simulink model "peacockElettricaSimulink"  (R2026a)
settings: Solver=FixedStepAuto  StopTime=40  FixedStep=0.001  EnableMultiTasking=on
InitFcn:
  | run('setupParams.m');
  | %run("tracks\track2.m");
StopFcn:
  | plot(out.X, out.Y);
  | axis equal;
  | grid on;
model workspace: external: MATLAB File (data not in the file)
values from neighbouring files (symbols this model uses):
  aero_bal_r = 0.5    [setupParams.m]    (also in setupParamsSingle.m)
  Af = 1.1    [setupParams.m]    (also in setupParamsSingle.m)
  auto_speed = 0    [setupParams.m]
  ay_limit = 15.0    (= 15)    [setupParams.m]    (also in setupParamsSingle.m)
  brake_bias_f = 0.40    (= 0.4)    [setupParams.m]    (also in setupParamsSingle.m = 0.6)
  brake_bias_r = 1 - brake_bias_f    (= 0.6)    [setupParams.m]    (also in setupParamsSingle.m = 0.4)
  camber_front = -1.5    [setupParams.m]    (also in setupParamsSingle.m)
  camber_rear = -1    [setupParams.m]    (also in setupParamsSingle.m)
  Cl = 1.0    (= 1)    [setupParams.m]    (also in setupParamsSingle.m)
  deathzone_APP = 5    [setupParams.m]    (also in setupParamsSingle.m)
  e_yaw_deadzone = 0.03    [setupParams.m]
  falling_slew_rate_torque = -500    [setupParams.m]    (also in setupParamsSingle.m)
  g = 9.81    [setupParams.m]    (also in setupParamsSingle.m)
  gnd_displ = 0.0    (= 0)    [setupParams.m]    (also in setupParamsSingle.m)
  h_o = 0.35    [setupParams.m]    (also in setupParamsSingle.m)
  I_charge_max = 21    [setupParams.m]
  I_discharge_max = 90    [setupParams.m]
  K_roll_rear = 0.6    [setupParams.m]    (also in setupParamsSingle.m = 0.5)
  Kus = 0.03    [setupParams.m]    (also in setupParamsSingle.m = 0)
  l_f = 0.775    [setupParams.m]    (also in setupParamsSingle.m)
  l_r = 0.775    [setupParams.m]    (also in setupParamsSingle.m)
  launch_ramp_rate = 1000.0    (= 1000)    [setupParams.m]    (also in setupParamsSingle.m)
  launch_V_thresh = 5.0    (= 5)    [setupParams.m]    (also in setupParamsSingle.m)
  mass = 320    [setupParams.m]    (also in setupParamsSingle.m = 300)
  mu = 1.5    [setupParams.m]    (also in setupParamsSingle.m)
  nominal_ramp_rate = 1000.0    (= 1000)    [setupParams.m]    (also in setupParamsSingle.m)
  overslip_factor = 1.01    [setupParams.m]    (also in setupParamsSingle.m = 1.13)
  pa_front_wheel = 82700    [setupParams.m]    (also in setupParamsSingle.m)
  pa_rear_wheel = 82700    [setupParams.m]    (also in setupParamsSingle.m)
  pedal_bp = (0:10:100)'    [setupParams.m]    (also in setupParamsSingle.m)
  pedal_map = (pedal_bp / 100) .^ pedal_alpha    [setupParams.m]    (also in setupParamsSingle.m = (pedal_bp / 100) .^ pedal_alpha.Value)
  R_wheel = 0.2032    [setupParams.m]    (also in setupParamsSingle.m)
  regen_I_cont_A = 14.0    (= 14)    [setupParams.m]    (also in setupParamsSingle.m)
  regen_I_peak_A = 21.0    (= 21)    [setupParams.m]    (also in setupParamsSingle.m)
  regen_I_peak_dur_s = 4.0    (= 4)    [setupParams.m]    (also in setupParamsSingle.m)
  regen_P_batt_max_W = 35000    [setupParams.m]    (also in setupParamsSingle.m)
  regen_pedal_thr = 5.0    (= 5)    [setupParams.m]    (also in setupParamsSingle.m = 10)
  regen_speed_crit_rpm = 1000    [setupParams.m]    (also in setupParamsSingle.m = 500)
  regen_speed_min_rpm = 4000    [setupParams.m]    (also in setupParamsSingle.m = 3000)
  regen_T_max = 9    [setupParams.m]    (also in setupParamsSingle.m = Simulink.Parameter(T_rated.Value/2))
  rho = 1.225    [setupParams.m]    (also in setupParamsSingle.m)
  rid_eff = 0.80    (= 0.8)    [setupParams.m]    (also in setupParamsSingle.m)
  rid_ratio = 15    [setupParams.m]    (also in setupParamsSingle.m)
  rising_slew_rate_torque = 100    [setupParams.m]    (also in setupParamsSingle.m)
  rpm_safe_threshold = 100    [setupParams.m]
  scale_factor_front = ones(27, 1)    [setupParams.m]    (also in setupParamsSingle.m)
  scale_factor_rear = ones(27, 1)    [setupParams.m]    (also in setupParamsSingle.m)
  slip_bc_coeff = 10    [setupParams.m]    (also in setupParamsSingle.m = Simulink.Parameter(1.5))
  slip_filt_N = 80    [setupParams.m]    (also in setupParamsSingle.m = 15)
  slip_Kd = 0.8    [setupParams.m]    (also in setupParamsSingle.m = Simulink.Parameter(5.0))
  slip_Ki = 13.0    (= 13)    [setupParams.m]    (also in setupParamsSingle.m = Simulink.Parameter(110.0))
  slip_Kp = 50.0    (= 50)    [setupParams.m]    (also in setupParamsSingle.m = Simulink.Parameter(180.0))
  slip_low_sat = 0.0    (= 0)    [setupParams.m]    (also in setupParamsSingle.m)
  slip_ref = 0.15    [setupParams.m]    (also in setupParamsSingle.m = Simulink.Parameter(0.15))
  slip_up_sat = 25    [setupParams.m]    (also in setupParamsSingle.m = 21)
  slip_V_min = 3    [setupParams.m]    (also in setupParamsSingle.m = 1)
  steer_ratio = 4.2    [pure_pursuit.m]    (also in setupParams.m; setupParamsSingle.m)
  steering_deadband = 1    [setupParams.m]
  T_headroom_k = 13.0    (= 13)    [setupParams.m]    (also in setupParamsSingle.m = Simulink.Parameter(5.0))
  T_headroom_max = 9    [setupParams.m]    (also in setupParamsSingle.m = Simulink.Parameter(5.0))
  T_peak = 20    [setupParams.m]    (also in setupParamsSingle.m = 21)
  T_rated = 9.8    [setupParams.m]    (also in setupParamsSingle.m = Simulink.Parameter(9.8))
  track_width = (track_width_r + track_width_f)/2    (= 1.2)    [setupParams.m]    (also in setupParamsSingle.m = sqrt(track_width_r^2 + track_width_f^2))
  track_width_f = 1.2    [setupParams.m]    (also in setupParamsSingle.m)
  track_width_r = 1.2    [setupParams.m]    (also in setupParamsSingle.m)
  Ts = 0.01    [setupParams.m]    (also in setupParamsSingle.m)
  tvc_bc = 17    [setupParams.m]
  tvc_D_thresh = 0.060    (= 0.06)    [setupParams.m]    (also in setupParamsSingle.m)
  tvc_D_thresh_off = 0.03    [setupParams.m]    (also in setupParamsSingle.m)
  tvc_Kd = 100    [setupParams.m]    (also in setupParamsSingle.m = Simulink.Parameter(5))
  tvc_Ki = 150    [setupParams.m]    (also in setupParamsSingle.m = Simulink.Parameter(10))
  tvc_Kp = 650    [setupParams.m]    (also in setupParamsSingle.m = Simulink.Parameter(70))
  tvc_N_filter = 25    [setupParams.m]    (also in setupParamsSingle.m = Simulink.Parameter(20))
  tvc_sat_dMz = 700    [setupParams.m]    (also in setupParamsSingle.m = Simulink.Parameter(10.0))
  tvc_throttle_on = 3.0    (= 3)    [setupParams.m]    (also in setupParamsSingle.m = Simulink.Parameter(3.0))
  tvc_tr = 5    [setupParams.m]    (also in setupParamsSingle.m = Simulink.Parameter(1.0))
  tvc_V_off = 2.0    (= 2)    [setupParams.m]    (also in setupParamsSingle.m = Simulink.Parameter(2.0))
  tvc_V_on = 4.0    (= 4)    [setupParams.m]    (also in setupParamsSingle.m = Simulink.Parameter(4.0))
  tvc_yaw_thresh = 0.08    [setupParams.m]    (also in setupParamsSingle.m)
  tvc_yaw_thresh_off = 0.04    [setupParams.m]    (also in setupParamsSingle.m)
  V_dc = 540    [setupParams.m]    (also in setupParamsSingle.m)
  w_engine = 0.005    [setupParams.m]    (also in setupParamsSingle.m)
  wheelbase = l_f + l_r    (= 1.55)    [setupParams.m]    (also in setupParamsSingle.m)
undefined symbols (not defined in the file or in its folder): V_ref, X_ref, Y_ref
libraries: simulink x74, slpidlib x8, vehdynlibtire x8, dspsigops x4, vehdynlibsteering x2, autolibshared x2, sim3dautolib x2, sim3dlib x1, robotalgslib x1
(part 1 of 6)
settings Model: SimulationMode=accelerator  SILPILModeSetting=veronly  ExtModeTrigDuration=10  Creator=Utente  LastModifiedBy=Utente
settings SolverCC: ZeroCrossControl=DisableAll  PositivePriorityOrder=on  EnableFixedStepZeroCrossing=on
settings DataIOCC: SaveFormat=StructureWithTime
settings OptimizationCC: BufferReuse=off
settings DebuggingCC: AlgebraicLoopMsg=error  MultiTaskRateTransMsg=warning
settings HardwareCC: ProdLargestAtomicInteger=Long  ProdLargestAtomicFloat=Double  ProdHWDeviceType=ARM Compatible->ARM Cortex-M  TargetLargestAtomicInteger=Long  TargetLargestAtomicFloat=Float  TargetIntDivRoundTo=Zero  TargetEndianess=LittleEndian  TargetHWDeviceType=ARM Compatible->ARM 10
settings ModelReferenceCC: ModelReferenceNumInstancesAllowed=Single
settings RTWCC: SystemTargetFile=ert.tlc  HardwareBoard=STM32G4xx Based  TLCOptions=-aInlineSetEventsForThisBaseRateFcn=TLC_FALSE -aSuppressMultiTaskScheduler=TLC_FALSE -aRateBasedStepFcn=1  GenCodeOnly=on  Toolchain=GNU Tools for STM32  BuildConfiguration=Faster Runs  Description=Embedded Coder
settings ERTTargetCC: ExtModeTransport=3.0  ExtModeStaticAllocSize=2048.0  CodeReplacementLibrary=ARM Cortex-M  SubcomponentCodeInterfacePackaging=Nonreusable function

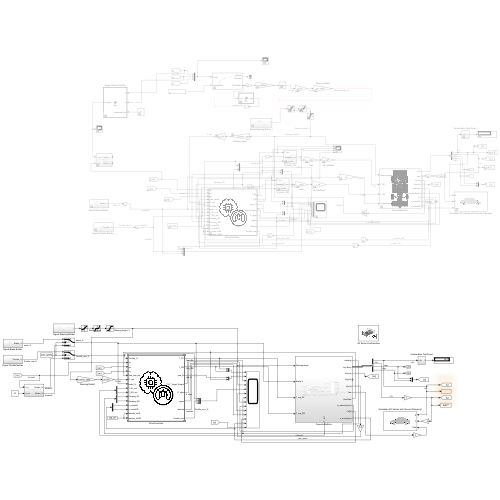
[thumbnail: Simulink's stored preview of the top-level diagram]
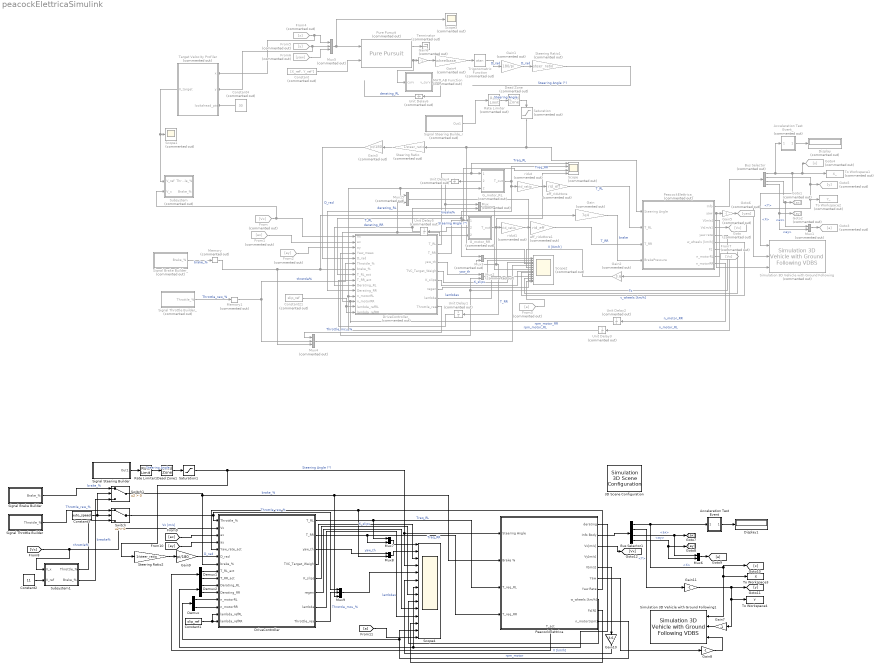
== system peacockElettricaSimulink ==
  " 3D Scene Configuration" : sim3dlib/Simulation 3D Scene Configuration  Priority=0  ProjectFormat=Default Scenes  SceneDesc=Open surface  ProjectName=Z:\.Programmi\MATLAB26a\toolbox\shared\sim3d_projects\automotive_project_windows\UE\WindowsNoEditor\VehicleSimulation.exe  ScenePath=/Game/Maps/HwStrght  EnableOpenDRIVE=off  vehTagList={'Custom';'Scene Origin';'SimulinkVehicle1';'SimulinkVehicle2'}  vehTag=SimulinkVehicle2  AttachedCameraRelativeTranslation=[0 0 0]  FreeCameraDefaultInitialTranslation=[-6, 0, 2]  AttachedCameraRelativeRotation=[0 0 0]  FreeCameraDefaultInitialRotation=[0, -15, 0]  ViewpointName=Custom  FreeCameraInitialTranslation=[0 0 0]  FreeCameraInitialRotation=[0 0 0]  OpVisEn=off  Ts=.03  EnableWindow=off  EnableRemoteAccess=off  SimulationMode=CoSimulation  SimulateUsing=Interpreted execution  EnableAnimationRecording=off  OverrideDefaultRecording=off  AnimationRecordingFileName=sim3dAnimation.mat  AnimationRecordingInterval=[0 inf]  EnableWeather=off  SunAzimuth=90  SunAltitude=40.0  EnableGeospatialSun=off  Latitude=0  Longitude=0  Date=2023-01-01  Time=10:30:00  GeoTimeZone=-5.0  SunDaylightSaving=off  wind=1  clouds=10  EnableVolumetricClouds=off  CloudCoverage=0  CloudAltitude=6  fog=0  rain=0  RaindropsEffect=off  SnowDensity=0  EnableGeospatial=off  TilesetSource=Earth terrain  UseTrueOrigin=off  OriginHeight=200  OriginLatitude=40.744652  OriginLongitude=-73.988864  MapStyle=Aerial  AdditionalAssetIDs=[]  UseAdvancedSunSky=off  SolarTime=11  TimeZone=-5  Day=21  Month=9  Year=2022  UseDaylightSavingTime=on  DSTStartDay=10  DSTStartMonth=3  DSTEndDay=3  DSTEndMonth=11  DSTSwitchHour=2  sensorTag=MainCamera1  sensorId=1  sensorName=MainCamera1  mountLoc=Origin  offsetFlag=off  tmountOffset=[0, 0, 0]  rmountOffset=[0, 0, 0]  HorizontalResolution=1280  VerticalResolution=720  HorizontalFOV=60  mountPoint=[0 0 0]  mountOrientation=[0 0 0]  aMode=2  ID=1  GeoTrigger=Inactive  ViewNameList={'Custom'}  ViewTranslationList={'[0 0 0]'}  ViewRotationList={'[0 0 0]'}
      settings: LibrarySourceBlock=vehdynlibsim3dcore/Simulation 3D Scene Configuration
  Acceleration Test Event : Subsystem
  Acceleration Test Event_ : Subsystem  Commented=on
  Bus Selector : BusSelector  Commented=on  OutputSignals=InertFrm.Geom.Disp.X,InertFrm.Geom.Disp.Y,BdyFrm.Cg.Acc.ax,BdyFrm.Cg.Acc.ay
  Bus Selector1 : BusSelector  OutputSignals=InertFrm.Geom.Disp.X,InertFrm.Geom.Disp.Y,BdyFrm.Cg.Acc.ax,BdyFrm.Cg.Acc.ay
  Constant : Constant  Commented=on  Value=[X_ref', Y_ref']
  Constant1 : Constant  Value=slip_ref
  Constant2 : Constant  Value=11
  Constant21 : Constant  Commented=on  Value=slip_ref
  Constant3 : Constant  Value=auto_speed
  Constant4 : Constant  Commented=on  Value=30
  Dead Zone : DeadZone  Commented=on  LowerValue=-2  UpperValue=2
  Dead Zone1 : DeadZone  LowerValue=-2  UpperValue=2
  Demux : Demux  Outputs=2
  Demux1 : Demux  Outputs=2
  Demux2 : Demux  Outputs=2
  Display : Display  Commented=on
  Display1 : Display
  DriveController : Subsystem  TreatAsAtomicUnit=on
      mask Display: image('smart_14958016.png', [0,0,0,0,60,60]);
  DriveController_ : Subsystem  Commented=on  TreatAsAtomicUnit=on
      mask Display: image('smart_14958016.png', [0,0,0,0,60,60]);
  From : From  Commented=on  GotoTag=Vx
  From1 : From  Commented=on  GotoTag=ax
  From2 : From  Commented=on  GotoTag=ay
  From3 : From  Commented=on  GotoTag=a
  From4 : From  Commented=on  GotoTag=x
  From5 : From  Commented=on  GotoTag=y
  From6 : From  Commented=on  GotoTag=yaw
  From7 : From  Commented=on  GotoTag=Vx
  G_motor_RL : Subsystem  Commented=on
      settings: PortSchema="{\"entries\":[{\"content\":{\"sides\":[{\"content\":{\"connectorIds\":[\"In1\",\"Out2\",\"In2\"]},\"type\":\"ConnectorPlacement.EquallySpacedRectSide\",\"uuid\":\"2f848e13-22e7-46a8-96e7-944fd1b36019\"},{\"content\":{\"connectorIds\":[\"Out1\"],\"side\":\"RIGHT\"},\"type\":\"ConnectorPlacement.EquallySpacedRectSide\",\"uuid\":\"64718f6e-925f-4c2e-9ed1-674a318236f8\"},{\"content\":{\"side\":\"TOP\"},\"type\":\"ConnectorPlacement.EquallySpacedRectSide\",\"uuid\":\"f53d168c-fae3-4286-a18b-c9c25d6ee575\"}]},\"type\":\"ConnectorPlacement.EquallySpacedConnector\",\"uuid\":\"bc8637a2-640e-4920-833f-efe601435780\"}],\"packageUris\":[\"http://schema.mathworks.com/mf0/Connector/R2020b\"],\"version\":\"1.0\"}"
  G_motor_RR : Subsystem  Commented=on
      settings: PortSchema="{\"entries\":[{\"content\":{\"sides\":[{\"content\":{\"connectorIds\":[\"In1\",\"Out2\",\"In2\"]},\"type\":\"ConnectorPlacement.EquallySpacedRectSide\",\"uuid\":\"b35581c9-4812-43f6-acf6-85982729658e\"},{\"content\":{\"connectorIds\":[\"Out1\"],\"side\":\"RIGHT\"},\"type\":\"ConnectorPlacement.EquallySpacedRectSide\",\"uuid\":\"46b9f9af-9e32-4108-a19f-3f2988ef12f0\"},{\"content\":{\"side\":\"TOP\"},\"type\":\"ConnectorPlacement.EquallySpacedRectSide\",\"uuid\":\"065300c1-2443-4807-8b2c-2500fecbac33\"}]},\"type\":\"ConnectorPlacement.EquallySpacedConnector\",\"uuid\":\"282786dd-8e40-401f-94f1-60a6482c0151\"}],\"packageUris\":[\"http://schema.mathworks.com/mf0/Connector/R2020b\"],\"version\":\"1.0\"}"
  Gain : Gain  Commented=on  Gain=7e4
  Gain1 : Gain  Commented=on  Gain=180/pi
  Gain10 : Gain  Gain=3.6
  Gain11 : Gain  Gain=-1
  Gain2 : Gain  Commented=on  Gain=3.6
  Gain3 : Gain  Commented=on  Gain=pi/180
  Gain4 : Gain  Commented=on  Gain=wheelbase
  Gain5 : Gain  Commented=on  Gain=-1
  Gain6 : Gain  Commented=on  Gain=-1
  Gain7 : Gain  Gain=-1
  Gain8 : Gain  Gain=-1
  Gain9 : Gain  Gain=pi/180
  Goto : Goto  Commented=on  GotoTag=Vx
  Goto1 : Goto  Commented=on  GotoTag=ax
  Goto2 : Goto  Commented=on  GotoTag=ay
  Goto3 : Goto  Commented=on  GotoTag=a
  Goto4 : Goto  Commented=on  GotoTag=x
  Goto5 : Goto  Commented=on  GotoTag=y
  Goto6 : Goto  Commented=on  GotoTag=yaw
  MATLAB Function : MATLAB Function  Commented=on  TreatAsAtomicUnit=on
  Memory : Memory  Commented=on
  Memory1 : Memory  Commented=on
  Mux{,1..3,15} (5 alike) : Mux  Commented=on  Inputs=2
  Mux4 : Mux  Commented=on  Inputs=3
  Mux5 : Mux  Commented=on  Inputs=3
  Mux6 : Mux  Inputs=2
  Mux7 : Mux  Inputs=2
  Mux8 : Mux  Inputs=2
  Mux9 : Mux  Inputs=3
  PeacockElettrica : Subsystem
      settings: PortSchema="{\"entries\":[{\"content\":{\"sides\":[{\"content\":{\"connectorIds\":[\"In1\",\"In2\",\"In3\",\"In4\"]},\"type\":\"ConnectorPlacement.EquallySpacedRectSide\",\"uuid\":\"9482d8e6-6871-478e-8a9d-73044ed7ab0e\"},{\"content\":{\"connectorIds\":[\"Out1\",\"Out2\",\"Out3\",\"Out4\",\"Out5\",\"Out6\",\"Out7\",\"Out8\",\"Out9\",\"Out10\"],\"side\":\"RIGHT\"},\"type\":\"ConnectorPlacement.EquallySpacedRectSide\",\"uuid\":\"cce15458-935a-453b-a26c-3a0c8875c305\"},{\"content\":{\"side\":\"TOP\"},\"type\":\"ConnectorPlacement.EquallySpacedRectSide\",\"uuid\":\"47cf2278-8524-4513-ad68-abd8f65e3014\"},{\"content\":{\"connectorIds\":[\"Out11\"],\"side\":\"BOTTOM\"},\"type\":\"ConnectorPlacement.EquallySpacedRectSide\",\"uuid\":\"d42c0be2-8d27-4d2e-97e3-233d61a32782\"}]},\"type\":\"ConnectorPlacement.EquallySpacedConnector\",\"uuid\":\"48bc61f2-5937-4956-9c2e-81c9fcf139cd\"}],\"packageUris\":[\"http://schema.mathworks.com/mf0/Connector/R2020b\"],\"version\":\"1.0\"}"
  PeacockElettrica_ : Subsystem  Commented=on
      mask Display: image('car.png', [0,0,0,0,60,100]);
  Pure Pursuit : robotalgslib/Pure Pursuit  Commented=on  DesiredLinearVelocityPort=off  DesiredLinearVelocity=0.1  MaxCurvature=1.0  LookaheadDistancePort=off  LookaheadDistance=1.5  TargetDirPort=off  SimulateUsing=Code generation
      settings: LibrarySourceBlock=navlib/Control Algorithms/Pure Pursuit
  Rate Limiter : RateLimiter  Commented=on  RisingSlewLimit=150  FallingSlewLimit=-150  SampleTimeMode=inherited
  Rate Limiter1 : RateLimiter  RisingSlewLimit=150  FallingSlewLimit=-150  SampleTimeMode=inherited
  Saturation : Saturate  Commented=on  UpperLimit=130  LowerLimit=-130
  Saturation1 : Saturate  UpperLimit=130  LowerLimit=-130
  Scope : Scope  Commented=on  NumInputPorts=4
      settings: ActiveDisplayYMinimum=-1.6967488885152928  ActiveDisplayYMaximum=15.270739996637639  DataLoggingVariableName=ScopeData5
  Scope1 : Scope  Commented=on
      settings: ActiveDisplayYMinimum=14.39563708692528  ActiveDisplayYMaximum=39.921268336925294  DataLoggingVariableName=ScopeData3
  Scope2 : Scope  Commented=on  NumInputPorts=14
      settings: AxesScalingNumUpdates=20  ActiveDisplayYMinimum=-11.688915556246606  ActiveDisplayYMaximum=16.101237530940978  DataLoggingVariableName=ScopeData2
  Scope3 : Scope  Commented=on
      settings: DataLoggingVariableName=ScopeData6
  Scope4 : Scope  NumInputPorts=14
      settings: ActiveDisplayYMinimum=-2.909562920832391  ActiveDisplayYMaximum=18.107750958840505  DataLoggingVariableName=ScopeData7
  Signal Brake Builder : Subsystem
  Signal Brake Builder_ : Subsystem  Commented=on
  Signal Steering Builde_r : Subsystem  Commented=on
  Signal Steering Builder : Subsystem
  Signal Throttle Builder : Subsystem
  Signal Throttle Builder_ : Subsystem  Commented=on
  Simulation 3D Vehicle with Ground Following : sim3dautolib/Simulation 3D Vehicle with Ground Following VDBS  Priority=-1  Commented=on  PassVehMesh=Formula student vehicle  MeshPath=/MathWorksAutomotiveContent/Vehicles/Muscle/Meshes/SK_MuscleCar.SK_MuscleCar  TrackWidth=1.9  WheelBase=3  WheelRadius=0.35  VehColor=Red  CoordinateSystem=SAE  InitialPos=[0, 0, 0]  InitialRot=[0,0,0]  ActorName=SimulinkVehicle1  VehLightsControl=off  HeadlightColor=[ 1, 1, 1 ]  HighBeamIntensity=100000  LowBeamIntensity=60000  HighBeamConeAngle=1.22  LowBeamConeAngle=1.22  LeftHeadlightOrientation=[ 0, 0 ]  RightHeadlightOrientation=[ 0, 0 ]  BrakelightIntensity=200  ReverselightIntensity=500  SignallightIntensity=500  SignallightPeriod=1  SignalPulseWidth=50  SampleTime=-1  ActorType=SimulinkVehicle  ID=1  aMode=2  ActorTag=SimulinkVehicle1  CoordinateScheme=0
      settings: LibrarySourceBlock=vehdynlibsim3d/Simulation 3D Vehicle with Ground Following
  Simulation 3D Vehicle with Ground Following1 : sim3dautolib/Simulation 3D Vehicle with Ground Following VDBS  Priority=-1  PassVehMesh=Formula student vehicle  MeshPath=/MathWorksAutomotiveContent/Vehicles/Muscle/Meshes/SK_MuscleCar.SK_MuscleCar  TrackWidth=1.9  WheelBase=3  WheelRadius=0.35  VehColor=Red  CoordinateSystem=SAE  InitialPos=[0, 0, 0]  InitialRot=[0,0,0]  ActorName=SimulinkVehicle2  VehLightsControl=off  HeadlightColor=[ 1, 1, 1 ]  HighBeamIntensity=100000  LowBeamIntensity=60000  HighBeamConeAngle=1.22  LowBeamConeAngle=1.22  LeftHeadlightOrientation=[ 0, 0 ]  RightHeadlightOrientation=[ 0, 0 ]  BrakelightIntensity=200  ReverselightIntensity=500  SignallightIntensity=500  SignallightPeriod=1  SignalPulseWidth=50  SampleTime=-1  ActorType=SimulinkVehicle  ID=2  aMode=2  ActorTag=SimulinkVehicle2  CoordinateScheme=0
      settings: LibrarySourceBlock=vehdynlibsim3d/Simulation 3D Vehicle with Ground Following
  Steering Ratio : Gain  Commented=on  Gain=1/steer_ratio
  Steering Ratio1 : Gain  Commented=on  Gain=steer_ratio
  Steering Ratio2 : Gain  Gain=1/steer_ratio
  Subsystem : Subsystem  Commented=on
  Subsystem1 : Subsystem
  Switch : Switch  Criteria=u2 > Threshold  SaturateOnIntegerOverflow=off  InputSameDT=off
  Switch1 : Switch  Criteria=u2 > Threshold  SaturateOnIntegerOverflow=off  InputSameDT=off
  Target Velocity Profiler : MATLAB Function  Commented=on  TreatAsAtomicUnit=on
  Terminator : Terminator  Commented=on
  To Workspace1 : ToWorkspace  Commented=on  VariableName=X_  SampleTime=0.05
  To Workspace2 : ToWorkspace  Commented=on  VariableName=Y_  SampleTime=0.05
  To Workspace3 : ToWorkspace  VariableName=X  SampleTime=0.05
  To Workspace4 : ToWorkspace  VariableName=Y  SampleTime=0.05
  Trigonometric Function : Trigonometry  Commented=on  Operator=atan
  Unit Delay{1..6} (6 alike) : UnitDelay  Commented=on  SampleTime=-1
  eff_riduttore : Gain  Commented=on  Gain=rid_eff
  eff_riduttore1 : Gain  Commented=on  Gain=rid_eff
  ridut : Gain  Commented=on  Gain=rid_ratio
  ridut1 : Gain  Commented=on  Gain=rid_ratio
  wires:
  G_motor_RL/1(T_out) -> Scope/2, DriveController_/8(T_RL_act), Mux3/1, ridut/1  "T_RL"
  Rate Limiter/1 -> Dead Zone/1  "Steering Angle"
  Saturation/1 -> PeacockElettrica_/1(Steering Angle), Scope2/4, Steering Ratio/1  "Steering Angle (°)"
  DriveController_/2(T_RR) -> Scope/3, G_motor_RR/1(T_req)  "Treq_RR"
  Bus Selector/1 -> Simulation 3D Vehicle with Ground Following/1, Goto4/1, To Workspace1/1, Acceleration Test Event_/1(<X>)  "<X>"
  eff_riduttore/1 -> PeacockElettrica_/2(T_RL)  "T_RL"
  Mux3/1 -> Scope2/1
  ridut1/1 -> eff_riduttore1/1
  ridut/1 -> eff_riduttore/1
  Steering Ratio/1 -> Gain3/1
  Bus Selector/2 -> Goto5/1, Simulation 3D Vehicle with Ground Following/2, To Workspace2/1  "<Y>"
  Dead Zone/1 -> Saturation/1
  G_motor_RR/1(T_out) -> Scope/4, Unit Delay1/1, Mux3/2, ridut1/1  "T_RR"
  Mux2/1 -> Scope2/2
  eff_riduttore1/1 -> PeacockElettrica_/3(T_RR)  "T_RR"
  DriveController_/1(T_RL) -> Scope/1, G_motor_RL/1(T_req)  "Treq_RL"
  PeacockElettrica_/5(yaw rate) -> DriveController_/4(Yaw_meas), Mux2/2
  Trigonometric Function/1 -> Gain1/1  "D_rad"
  Unit Delay1/1 -> DriveController_/9(T_RR_act)
  Unit Delay5/1 -> Mux/2, DriveController_/10(Derating_RL)  "derating_RR"
  G_motor_RL/2(derating) -> Unit Delay4/1
  DriveController_/3(yaw_th) -> Mux2/1  "yaw_th"
  DriveController_/4(TVC_Target_Weight) -> Scope2/3
  Mux/1 -> Scope2/7
  Signal Throttle Builder_/1(Throttle_%) -> Memory1/1  "Throttle_raw_%"
  Mux4/1 -> Scope2/5
  Constant21/1 -> DriveController_/14(lambda_refRL), DriveController_/15(lambda_refRR)
  DriveController_/5(K_slips) -> Scope2/8  "K_slips"
  DriveController_/6(regen) -> Scope2/10
  DriveController_/8(Throttle_real) -> Mux4/1  "Throttle_mcu_%"
  DriveController_/7(lambda) -> Scope2/11  "lambdas"
  Unit Delay4/1 -> Mux/1, DriveController_/11(Derating_RR)  "derating_RL"
  G_motor_RR/2(derating) -> Unit Delay5/1
  Mux15/1 -> Scope2/13
  PeacockElettrica_/8(n_motorRL) -> Unit Delay3/1  "n_motor_RL"
  PeacockElettrica_/9(n_motorRR) -> Unit Delay2/1  "n_motor_RR"
  PeacockElettrica_/1(Info) -> Bus Selector/1
  PeacockElettrica_/2(yaw) -> Gain5/1, Simulation 3D Vehicle with Ground Following/3
  PeacockElettrica_/3(V[m/s]) -> Gain2/1
  PeacockElettrica_/6(w_wheels [km/h]) -> Scope2/9  "v_wheels [km/h]"
  PeacockElettrica_/7(Fz) -> Scope2/12  "Fz"
  Gain2/1 -> Scope2/6  "V [Km/h]"
  PeacockElettrica_/4(Vx[m/s]) -> Goto/1
  From/1 -> Subsystem/2(V_x), DriveController_/1(Vx)
  From1/1 -> DriveController_/2(ax)
  Bus Selector/4 -> Goto2/1, Mux1/2  "<ay>"
  Bus Selector/3 -> Mux1/1, Goto1/1  "<ax>"
  From2/1 -> DriveController_/3(ay)
  Signal Brake Builder_/1(Brake_%) -> Memory/1  "brake_%"
  Acceleration Test Event_/1(Out1) -> Display/1
  Mux1/1 -> Goto3/1
  From3/1 -> Scope2/14
  Unit Delay2/1 -> G_motor_RR/2(rpm_motor), Mux15/2, DriveController_/13(n_motorRR)  "rpm_motor_RR"
  Unit Delay3/1 -> Mux15/1, G_motor_RL/2(rpm_motor), DriveController_/12(n_motorRL)  "rpm_motor_RL"
  Signal Steering Builde_r/1(Out1) -> Rate Limiter/1
  Gain/1 -> PeacockElettrica_/4(BrakePressure)  "brake"
  Mux5/1 -> Scope3/1, Pure Pursuit/1
  From4/1 -> Target Velocity Profiler/1(x), Mux5/1
  From5/1 -> Target Velocity Profiler/2(y), Mux5/2
  From6/1 -> Mux5/3
  Gain4/1 -> Trigonometric Function/1
  Constant/1 -> Pure Pursuit/2
  Gain1/1 -> Steering Ratio1/1  "D_rad"
  Gain3/1 -> DriveController_/5(D_rad)  "D_rad"
  Memory/1 -> Gain/1, DriveController_/7(brake_%), Mux4/3  "breake%"
  Memory1/1 -> DriveController_/6(Throttle_%), Mux4/2  "throttle%"
  Steering Ratio1/1 -> ?  "Steering Angle (°)"
  MATLAB Function/1(v_curv) -> Unit Delay6/1
  Unit Delay6/1 -> ?  "derating_RL"
  Gain5/1 -> Goto6/1
  Constant4/1 -> Target Velocity Profiler/3(lookahead_pts)
  Target Velocity Profiler/1(V_target) -> Scope1/1, Subsystem/1(V_ref)
  Pure Pursuit/1 -> Terminator/1
  Pure Pursuit/2 -> Gain6/1, MATLAB Function/1(curv)
  Gain6/1 -> Gain4/1
  DriveController/1(T_RL) -> Mux7/1, PeacockElettrica/3(T_req_RL)  "Treq_RL"
  DriveController/2(T_RR) -> Mux7/2, PeacockElettrica/4(T_req_RR)  "Treq_RR"
  Switch1/1 -> DriveController/7(brake_%), PeacockElettrica/2(Brake %), Mux9/3  "brake_%"
  Signal Steering Builder/1(Out1) -> Rate Limiter1/1
  Rate Limiter1/1 -> Dead Zone1/1  "Steering Angle"
  Dead Zone1/1 -> Saturation1/1
  Switch/1 -> Mux9/1, DriveController/1(Throttle_%)  "Throttle_raw_%"
  PeacockElettrica/10(n_motor[rpm]) -> Scope4/13, Demux/1  "rpm_motor"
  Demux/1 -> DriveController/12(n_motorRL)
  Demux/2 -> DriveController/13(n_motorRR)
  Constant1/1 -> DriveController/14(lambda_refRL), DriveController/15(lambda_refRR)
  PeacockElettrica/2(Info Body) -> Bus Selector1/1
  Bus Selector1/3 -> Mux6/1, [ax]  "<ax>"
  Bus Selector1/4 -> Mux6/2, [ay]  "<ay>"
  Mux6/1 -> [a]
  Bus Selector1/2 -> Gain11/1  "<Y>"
  PeacockElettrica/6(Yaw) -> Gain8/1
  Gain7/1 -> Simulation 3D Vehicle with Ground Following1/2
  Gain8/1 -> Simulation 3D Vehicle with Ground Following1/3
  Acceleration Test Event/1(Out1) -> Display1/1
  Bus Selector1/1 -> Acceleration Test Event/1(<X>), Simulation 3D Vehicle with Ground Following1/1, To Workspace3/1, [x]  "<X>"
  PeacockElettrica/3(Vx[m/s]) -> [Vx]
  [Vx] -> Subsystem1/1(V_x), DriveController/2(Vx)  "Vx [m/s]"
  PeacockElettrica/11(T_act) -> Demux1/1
  Demux1/1 -> DriveController/8(T_RL_act)
  Demux1/2 -> DriveController/9(T_RR_act)
  PeacockElettrica/1(derating) -> Scope4/7, Demux2/1
  Demux2/1 -> DriveController/10(Derating_RL)
  Demux2/2 -> DriveController/11(Derating_RR)
  PeacockElettrica/7(Yaw Rate) -> Mux8/2, DriveController/5(Yaw_rate_act)
  Saturation1/1 -> Steering Ratio2/1, PeacockElettrica/1(Steering Angle), Scope4/4  "Steering Angle (°)"
  Steering Ratio2/1 -> Gain9/1
  Gain9/1 -> DriveController/6(D_rad)  "D_rad"
  [ax] -> DriveController/3(ax)
  [ay] -> DriveController/4(ay)
  Mux7/1 -> Scope4/1
  DriveController/3(yaw_th) -> Mux8/1  "yaw_th"
  Mux8/1 -> Scope4/2
  DriveController/4(TVC_Target_Weight) -> Scope4/3
  DriveController/8(Throttle_real) -> Mux9/2  "Throttle_mcu_%"
  Mux9/1 -> Scope4/5
  PeacockElettrica/5(V[m/s]) -> Gain10/1
  Gain10/1 -> Scope4/6  "V [km/h]"
  DriveController/5(K_slips) -> Scope4/8  "K_slips"
  PeacockElettrica/8(w_wheels [km/h]) -> Scope4/9
  DriveController/6(regen) -> Scope4/10
  DriveController/7(lambda) -> Scope4/11  "lambdas"
  PeacockElettrica/9(Fz[N]) -> Scope4/12
  [a] -> Scope4/14
  Gain11/1 -> Gain7/1, To Workspace4/1, [y]
  Constant2/1 -> Subsystem1/2(V_ref)
  Signal Throttle Builder/1(Throttle_%) -> Switch/1  "Throttle_raw_%"
  Signal Brake Builder/1(Brake_%) -> Switch1/1  "brake_%"
  Subsystem1/1(Throttle_%) -> Switch/3  "throttle%"
  Subsystem1/2(Brake_%) -> Switch1/3  "breake%"
  Constant3/1 -> Switch1/2, Switch/2

== system peacockElettricaSimulink/Acceleration Test Event ==
  <X> : Inport
  Clock : Clock
  Clock1 : Clock
  Finish : HitCross  HitCrossingOffset=75.3  HitCrossingDirection=rising
  Sample and Hold : dspsigops/Sample and Hold  trig=Rising edge  initCond=0  latchinput=off
  Sample and Hold1 : dspsigops/Sample and Hold  trig=Rising edge  initCond=0  latchinput=off
  Start : HitCross  HitCrossingOffset=0.3  HitCrossingDirection=rising
  Sum : Sum  Inputs=|-+
  Out1 : Outport
  wires:
  Sample and Hold/1 -> Sum/2
  Sample and Hold1/1 -> Sum/1
  Finish/1 -> Sample and Hold/Trigger
  <X>/1 -> Finish/1, Start/1
  Clock1/1 -> Sample and Hold1/1
  Start/1 -> Sample and Hold1/Trigger
  Sum/1 -> Out1/1
  Clock/1 -> Sample and Hold/1

== system peacockElettricaSimulink/Acceleration Test Event_ ==
  <X> : Inport
  Clock : Clock
  Clock1 : Clock
  Finish : HitCross  HitCrossingOffset=75.3  HitCrossingDirection=rising
  Sample and Hold : dspsigops/Sample and Hold  trig=Rising edge  initCond=0  latchinput=off
  Sample and Hold1 : dspsigops/Sample and Hold  trig=Rising edge  initCond=0  latchinput=off
  Start : HitCross  HitCrossingOffset=0.3  HitCrossingDirection=rising
  Sum : Sum  Inputs=|-+
  Out1 : Outport
  wires:
  Sample and Hold/1 -> Sum/2
  Sample and Hold1/1 -> Sum/1
  Finish/1 -> Sample and Hold/Trigger
  <X>/1 -> Finish/1, Start/1
  Clock1/1 -> Sample and Hold1/1
  Start/1 -> Sample and Hold1/Trigger
  Sum/1 -> Out1/1
  Clock/1 -> Sample and Hold/1

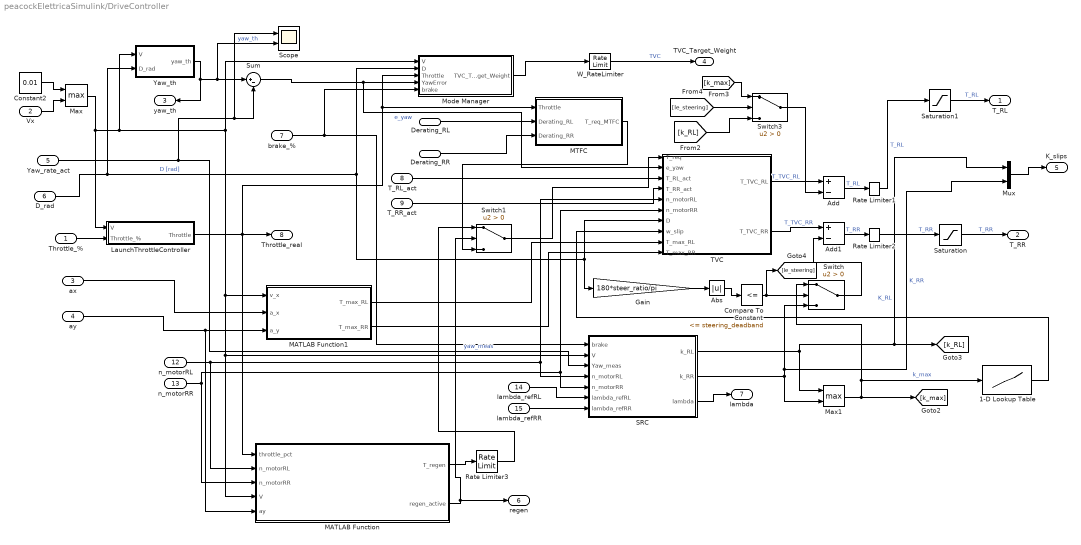
== system peacockElettricaSimulink/DriveController ==
  Throttle_% : Inport
  Vx : Inport  Port=2
  ax : Inport  Port=3
  ay : Inport  Port=4
  Yaw_rate_act : Inport  Port=5
  D_rad : Inport  Port=6
  brake_% : Inport  Port=7
  T_RL_act : Inport  Port=8
  T_RR_act : Inport  Port=9
  Derating_RL : Inport  Port=10
  Derating_RR : Inport  Port=11
  n_motorRL : Inport  Port=12
  n_motorRR : Inport  Port=13
  lambda_refRL : Inport  Port=14
  lambda_refRR : Inport  Port=15
  1-D Lookup Table : Lookup_n-D  NumberOfTableDimensions=1  BreakpointsForDimension1=[0,3,12]  Table=[1,1,0]  ExtrapMethod=Clip  UseLastTableValue=on  InternalRulePriority=Speed  RndMeth=Simplest
  Abs : Abs  SaturateOnIntegerOverflow=off
  Add : Sum  Inputs=+-
  Add1 : Sum  Inputs=+-
  Compare To Constant : simulink/Logic and Bit Operations/Compare To Constant  relop=<=  const=steering_deadband  OutDataTypeStr=boolean
  Constant2 : Constant  Value=0.01
  Gain : Gain  Gain=180*steer_ratio/pi
  LaunchThrottleController : Subsystem
  MATLAB Function : MATLAB Function  TreatAsAtomicUnit=on
  MATLAB Function1 : MATLAB Function  TreatAsAtomicUnit=on
  MTFC : Subsystem
  Max : MinMax  Function=max  Inputs=2
  Max1 : MinMax  Function=max  Inputs=2
  Mode Manager : Stateflow chart  TreatAsAtomicUnit=on
  Mux : Mux  Inputs=2
  Rate Limiter1 : RateLimiter  RisingSlewLimit=rising_slew_rate_torque  FallingSlewLimit=falling_slew_rate_torque  SampleTimeMode=inherited
  Rate Limiter2 : RateLimiter  RisingSlewLimit=rising_slew_rate_torque  FallingSlewLimit=falling_slew_rate_torque  SampleTimeMode=inherited
  Rate Limiter3 : RateLimiter  RisingSlewLimit=60  FallingSlewLimit=-20  SampleTimeMode=inherited
  SRC : Subsystem
  Saturation : Saturate  UpperLimit=T_peak  LowerLimit=-regen_T_max
  Saturation1 : Saturate  UpperLimit=T_peak  LowerLimit=-regen_T_max
  Scope : Scope  NumInputPorts=2
      settings: ActiveDisplayYMinimum=-1.2846466868170756  ActiveDisplayYMaximum=1.5088492229704735
  Sum : Sum  Inputs=|+-
  Switch : Switch  Criteria=u2 > Threshold  SaturateOnIntegerOverflow=off  InputSameDT=off
  Switch1 : Switch  Criteria=u2 > Threshold  SaturateOnIntegerOverflow=off  InputSameDT=off
  Switch3 : Switch  Criteria=u2 > Threshold  SaturateOnIntegerOverflow=off  InputSameDT=off
  TVC : Subsystem
  W_RateLimiter : RateLimiter  RisingSlewLimit=2  FallingSlewLimit=-2  SampleTimeMode=inherited
  Yaw_th : Subsystem
  T_RL : Outport
  T_RR : Outport  Port=2
  yaw_th : Outport  Port=3
  TVC_Target_Weight : Outport  Port=4
  K_slips : Outport  Port=5
  regen : Outport  Port=6
  lambda : Outport  Port=7
  Throttle_real : Outport  Port=8
  wires:
  D_rad/1 -> TVC/7(D), Gain/1, Mode Manager/2(D), Yaw_th/2(D_rad)  "D [rad]"
  Yaw_th/1(yaw_th) -> Scope/2, Sum/1, yaw_th/1  "yaw_th"
  Derating_RL/1 -> MTFC/2(Derating_RL)
  Yaw_rate_act/1 -> SRC/3(Yaw_meas), Scope/1, Sum/2  "yaw_meas"
  Derating_RR/1 -> MTFC/3(Derating_RR)
  TVC/2(T_TVC_RR) -> Add1/1  "T_TVC_RR"
  Max/1 -> LaunchThrottleController/1(V), MATLAB Function/4(V), SRC/2(V), MATLAB Function1/1(v_x), Mode Manager/1(V), Yaw_th/1(V)
  T_RL_act/1 -> TVC/3(T_RL_act)
  T_RR_act/1 -> TVC/4(T_RR_act)
  TVC/1(T_TVC_RL) -> Add/1  "T_TVC_RL"
  brake_%/1 -> SRC/1(brake), Mode Manager/5(brake)
  Sum/1 -> TVC/2(e_yaw), Mode Manager/4(YawError)  "e_yaw"
  W_RateLimiter/1 -> TVC_Target_Weight/1  "TVC"
  Add/1 -> Rate Limiter1/1  "T_RL"
  Add1/1 -> Rate Limiter2/1  "T_RR"
  n_motorRL/1 -> TVC/5(n_motorRL), SRC/4(n_motorRL), MATLAB Function/2(n_motorRL)
  n_motorRR/1 -> TVC/6(n_motorRR), SRC/5(n_motorRR), MATLAB Function/3(n_motorRR)
  lambda_refRL/1 -> SRC/6(lambda_refRL)
  lambda_refRR/1 -> SRC/7(lambda_refRR)
  SRC/1(k_RL) -> Mux/1, [k_RL], Max1/1  "K_RL"
  SRC/2(k_RR) -> Switch/3, Mux/2, Max1/2  "K_RR"
  Saturation/1 -> T_RR/1  "T_RR"
  Mux/1 -> K_slips/1
  MATLAB Function/1(T_regen) -> Rate Limiter3/1
  MATLAB Function/2(regen_active) -> Switch1/2, regen/1
  Saturation1/1 -> T_RL/1  "T_RL"
  Rate Limiter2/1 -> Saturation/1  "T_RR"
  Throttle_%/1 -> LaunchThrottleController/2(Throttle_%)
  SRC/3(lambda) -> lambda/1
  MATLAB Function1/1(T_max_RL) -> TVC/9(T_max_RL)
  ay/1 -> MATLAB Function/5(ay), MATLAB Function1/3(a_y)
  ax/1 -> MATLAB Function1/2(a_x)
  MATLAB Function1/2(T_max_RR) -> TVC/10(T_max_RR)
  Rate Limiter1/1 -> Saturation1/1  "T_RL"
  MTFC/1(T_req_MTFC) -> Switch1/3
  Vx/1 -> Max/2
  Constant2/1 -> Max/1
  Max1/1 -> 1-D Lookup Table/1, Switch/1, [k_max]  "k_max"
  Switch/1 -> Add1/2
  Gain/1 -> Abs/1
  Compare To Constant/1 -> [le_steering], Switch/2
  [k_RL] -> Switch3/3
  Switch3/1 -> Add/2
  [k_max] -> Switch3/1
  [le_steering] -> Switch3/2
  1-D Lookup Table/1 -> TVC/8(w_slip)
  Abs/1 -> Compare To Constant/1
  Rate Limiter3/1 -> Switch1/1
  Switch1/1 -> TVC/1(T_req)
  LaunchThrottleController/1(Throttle) -> MATLAB Function/1(throttle_pct), Mode Manager/3(Throttle), MTFC/1(Throttle), Throttle_real/1
  Mode Manager/1(TVC_Target_Weight) -> W_RateLimiter/1

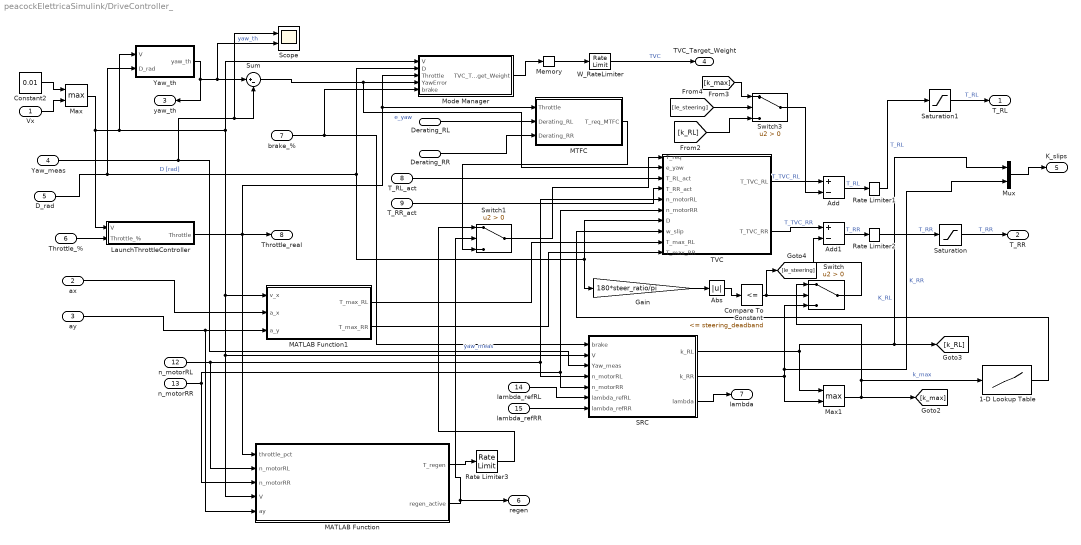
== system peacockElettricaSimulink/DriveController_ ==
  Vx : Inport
  ax : Inport  Port=2
  ay : Inport  Port=3
  Yaw_meas : Inport  Port=4
  D_rad : Inport  Port=5
  Throttle_% : Inport  Port=6
  brake_% : Inport  Port=7
  T_RL_act : Inport  Port=8
  T_RR_act : Inport  Port=9
  Derating_RL : Inport  Port=10
  Derating_RR : Inport  Port=11
  n_motorRL : Inport  Port=12
  n_motorRR : Inport  Port=13
  lambda_refRL : Inport  Port=14
  lambda_refRR : Inport  Port=15
  1-D Lookup Table : Lookup_n-D  NumberOfTableDimensions=1  BreakpointsForDimension1=[0,3,12]  Table=[1,1,0]  ExtrapMethod=Clip  UseLastTableValue=on  InternalRulePriority=Speed  RndMeth=Simplest
  Abs : Abs  SaturateOnIntegerOverflow=off
  Add : Sum  Inputs=+-
  Add1 : Sum  Inputs=+-
  Compare To Constant : simulink/Logic and Bit Operations/Compare To Constant  relop=<=  const=steering_deadband  OutDataTypeStr=boolean
  Constant2 : Constant  Value=0.01
  Gain : Gain  Gain=180*steer_ratio/pi
  LaunchThrottleController : Subsystem
  MATLAB Function : MATLAB Function  TreatAsAtomicUnit=on
  MATLAB Function1 : MATLAB Function  TreatAsAtomicUnit=on
  MTFC : Subsystem
  Max : MinMax  Function=max  Inputs=2
  Max1 : MinMax  Function=max  Inputs=2
  Memory : Memory
  Mode Manager : Stateflow chart  TreatAsAtomicUnit=on
  Mux : Mux  Inputs=2
  Rate Limiter1 : RateLimiter  RisingSlewLimit=rising_slew_rate_torque  FallingSlewLimit=falling_slew_rate_torque  SampleTimeMode=inherited
  Rate Limiter2 : RateLimiter  RisingSlewLimit=rising_slew_rate_torque  FallingSlewLimit=falling_slew_rate_torque  SampleTimeMode=inherited
  Rate Limiter3 : RateLimiter  RisingSlewLimit=60  FallingSlewLimit=-20  SampleTimeMode=inherited
  SRC : Subsystem
  Saturation : Saturate  UpperLimit=T_peak  LowerLimit=-regen_T_max
  Saturation1 : Saturate  UpperLimit=T_peak  LowerLimit=-regen_T_max
  Scope : Scope  NumInputPorts=2
      settings: ActiveDisplayYMinimum=-1.2846466868170756  ActiveDisplayYMaximum=1.5088492229704735
  Sum : Sum  Inputs=|+-
  Switch : Switch  Criteria=u2 > Threshold  SaturateOnIntegerOverflow=off  InputSameDT=off
  Switch1 : Switch  Criteria=u2 > Threshold  SaturateOnIntegerOverflow=off  InputSameDT=off
  Switch3 : Switch  Criteria=u2 > Threshold  SaturateOnIntegerOverflow=off  InputSameDT=off
  TVC : Subsystem
  W_RateLimiter : RateLimiter  RisingSlewLimit=2  FallingSlewLimit=-2  SampleTimeMode=inherited
  Yaw_th : Subsystem
  T_RL : Outport
  T_RR : Outport  Port=2
  yaw_th : Outport  Port=3
  TVC_Target_Weight : Outport  Port=4
  K_slips : Outport  Port=5
  regen : Outport  Port=6
  lambda : Outport  Port=7
  Throttle_real : Outport  Port=8
  wires:
  D_rad/1 -> TVC/7(D), Gain/1, Mode Manager/2(D), Yaw_th/2(D_rad)  "D [rad]"
  Yaw_th/1(yaw_th) -> Scope/2, Sum/1, yaw_th/1  "yaw_th"
  Derating_RL/1 -> MTFC/2(Derating_RL)
  Yaw_meas/1 -> SRC/3(Yaw_meas), Scope/1, Sum/2  "yaw_meas"
  Derating_RR/1 -> MTFC/3(Derating_RR)
  TVC/2(T_TVC_RR) -> Add1/1  "T_TVC_RR"
  Max/1 -> LaunchThrottleController/1(V), MATLAB Function/4(V), SRC/2(V), MATLAB Function1/1(v_x), Mode Manager/1(V), Yaw_th/1(V)
  T_RL_act/1 -> TVC/3(T_RL_act)
  T_RR_act/1 -> TVC/4(T_RR_act)
  TVC/1(T_TVC_RL) -> Add/1  "T_TVC_RL"
  brake_%/1 -> SRC/1(brake), Mode Manager/5(brake)
  Sum/1 -> TVC/2(e_yaw), Mode Manager/4(YawError)  "e_yaw"
  W_RateLimiter/1 -> TVC_Target_Weight/1  "TVC"
  Mode Manager/1(TVC_Target_Weight) -> Memory/1
  Add/1 -> Rate Limiter1/1  "T_RL"
  Add1/1 -> Rate Limiter2/1  "T_RR"
  n_motorRL/1 -> TVC/5(n_motorRL), SRC/4(n_motorRL), MATLAB Function/2(n_motorRL)
  n_motorRR/1 -> TVC/6(n_motorRR), SRC/5(n_motorRR), MATLAB Function/3(n_motorRR)
  lambda_refRL/1 -> SRC/6(lambda_refRL)
  lambda_refRR/1 -> SRC/7(lambda_refRR)
  SRC/1(k_RL) -> Mux/1, [k_RL], Max1/1  "K_RL"
  SRC/2(k_RR) -> Switch/3, Mux/2, Max1/2  "K_RR"
  Saturation/1 -> T_RR/1  "T_RR"
  Mux/1 -> K_slips/1
  MATLAB Function/1(T_regen) -> Rate Limiter3/1
  MATLAB Function/2(regen_active) -> Switch1/2, regen/1
  Saturation1/1 -> T_RL/1  "T_RL"
  Rate Limiter2/1 -> Saturation/1  "T_RR"
  Throttle_%/1 -> LaunchThrottleController/2(Throttle_%)
  SRC/3(lambda) -> lambda/1
  MATLAB Function1/1(T_max_RL) -> TVC/9(T_max_RL)
  ay/1 -> MATLAB Function/5(ay), MATLAB Function1/3(a_y)
  ax/1 -> MATLAB Function1/2(a_x)
  MATLAB Function1/2(T_max_RR) -> TVC/10(T_max_RR)
  Rate Limiter1/1 -> Saturation1/1  "T_RL"
  MTFC/1(T_req_MTFC) -> Switch1/3
  Vx/1 -> Max/2
  Constant2/1 -> Max/1
  Max1/1 -> 1-D Lookup Table/1, Switch/1, [k_max]  "k_max"
  Switch/1 -> Add1/2
  Gain/1 -> Abs/1
  Compare To Constant/1 -> [le_steering], Switch/2
  [k_RL] -> Switch3/3
  Switch3/1 -> Add/2
  [k_max] -> Switch3/1
  [le_steering] -> Switch3/2
  1-D Lookup Table/1 -> TVC/8(w_slip)
  Abs/1 -> Compare To Constant/1
  Rate Limiter3/1 -> Switch1/1
  Switch1/1 -> TVC/1(T_req)
  LaunchThrottleController/1(Throttle) -> MATLAB Function/1(throttle_pct), Mode Manager/3(Throttle), MTFC/1(Throttle), Throttle_real/1
  Memory/1 -> W_RateLimiter/1

== system peacockElettricaSimulink/G_motor_RL ==
  T_req : Inport
  rpm_motor : Inport  Port=2
  1-D Lookup Table : Lookup_n-D  NumberOfTableDimensions=1  BreakpointsForDimension1=[0, 9268, 11586.6]  Table=[21, 21, 9.8]  InternalRulePriority=Speed  RndMeth=Simplest
  Constant : Constant  Value=V_dc
  Derating : MATLAB Function  TreatAsAtomicUnit=on
  Field weakening : MATLAB Function  TreatAsAtomicUnit=on
  Gain : Gain  Gain=1/0.26
  I_n ^2 : Constant  Value=1681
  Integrator : Integrator  LimitOutput=on  UpperSaturationLimit=11586.6  LowerSaturationLimit=0
  Math Function : Math  Operator=square
  Min : MinMax  Inputs=3
  Sum : Sum  Inputs=|+-
  Transfer Fcn : TransferFcn  Denominator=[w_engine 1]
  Unit Delay : UnitDelay  SampleTime=-1
  T_out : Outport
  derating : Outport  Port=2
  wires:
  Sum/1 -> Integrator/1
  I_n ^2/1 -> Sum/2
  Gain/1 -> Math Function/1  "I_req"
  Math Function/1 -> Sum/1
  Integrator/1 -> 1-D Lookup Table/1
  Min/1 -> Transfer Fcn/1
  Transfer Fcn/1 -> T_out/1
  1-D Lookup Table/1 -> Derating/1(T_thermal), Min/1  "T_thermal_limit"
  Derating/1(derating_out) -> Unit Delay/1, derating/1
  Unit Delay/1 -> Derating/3(derating_prev)
  rpm_motor/1 -> Field weakening/1(rpm_motor)
  Field weakening/1(T_limit) -> Min/3
  T_req/1 -> Derating/2(T_req), Gain/1, Min/2
  Constant/1 -> Field weakening/2(V_dc)

== system peacockElettricaSimulink/G_motor_RR ==
  T_req : Inport
  rpm_motor : Inport  Port=2
  1-D Lookup Table : Lookup_n-D  NumberOfTableDimensions=1  BreakpointsForDimension1=[0, 9268, 11586.6]  Table=[21, 21, 9.8]  InternalRulePriority=Speed  RndMeth=Simplest
  Constant : Constant  Value=V_dc
  Gain : Gain  Gain=1/0.26
  I_n ^2 : Constant  Value=1681
  Integrator : Integrator  LimitOutput=on  UpperSaturationLimit=11586.6  LowerSaturationLimit=0
  MATLAB Function : MATLAB Function  TreatAsAtomicUnit=on
  MATLAB Function1 : MATLAB Function  TreatAsAtomicUnit=on
  Math Function : Math  Operator=square
  Min : MinMax  Inputs=3
  Sum : Sum  Inputs=|+-
  Transfer Fcn : TransferFcn  Denominator=[w_engine 1]
  Unit Delay : UnitDelay  SampleTime=-1
  T_out : Outport
  derating : Outport  Port=2
  wires:
  Sum/1 -> Integrator/1
  MATLAB Function/1(derating_out) -> Unit Delay/1, derating/1
  Unit Delay/1 -> MATLAB Function/3(derating_prev)
  Integrator/1 -> 1-D Lookup Table/1
  T_req/1 -> MATLAB Function/2(T_req), Gain/1, Min/2
  Math Function/1 -> Sum/1
  Transfer Fcn/1 -> T_out/1
  Gain/1 -> Math Function/1  "I_req"
  I_n ^2/1 -> Sum/2
  rpm_motor/1 -> MATLAB Function1/1(rpm_motor)
  MATLAB Function1/1(T_limit) -> Min/3
  1-D Lookup Table/1 -> MATLAB Function/1(T_thermal), Min/1  "T_thermal_limit"
  Min/1 -> Transfer Fcn/1
  Constant/1 -> MATLAB Function1/2(V_dc)

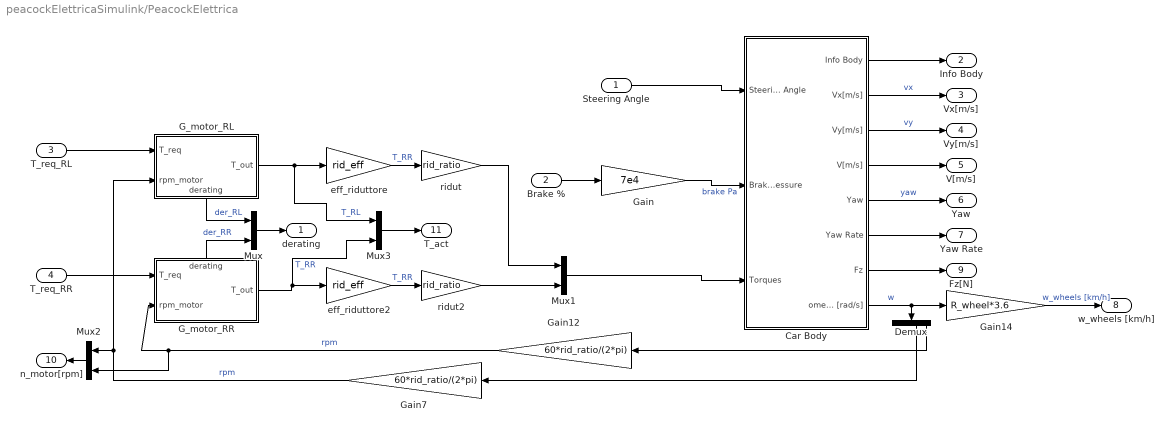
== system peacockElettricaSimulink/PeacockElettrica ==
  Steering Angle : Inport
  Brake % : Inport  Port=2
  T_req_RL : Inport  Port=3
  T_req_RR : Inport  Port=4
  Car Body : Subsystem
  Demux : Demux
  G_motor_RL : Subsystem
      settings: PortSchema="{\"entries\":[{\"content\":{\"sides\":[{\"content\":{\"connectorIds\":[\"In1\",\"In2\"]},\"type\":\"ConnectorPlacement.EquallySpacedRectSide\",\"uuid\":\"2f848e13-22e7-46a8-96e7-944fd1b36019\"},{\"content\":{\"connectorIds\":[\"Out1\"],\"side\":\"RIGHT\"},\"type\":\"ConnectorPlacement.EquallySpacedRectSide\",\"uuid\":\"64718f6e-925f-4c2e-9ed1-674a318236f8\"},{\"content\":{\"side\":\"TOP\"},\"type\":\"ConnectorPlacement.EquallySpacedRectSide\",\"uuid\":\"f53d168c-fae3-4286-a18b-c9c25d6ee575\"},{\"content\":{\"connectorIds\":[\"Out2\"],\"side\":\"BOTTOM\"},\"type\":\"ConnectorPlacement.EquallySpacedRectSide\",\"uuid\":\"aa9b5dac-f6fd-4716-b4b4-21a792f168ed\"}]},\"type\":\"ConnectorPlacement.EquallySpacedConnector\",\"uuid\":\"bc8637a2-640e-4920-833f-efe601435780\"}],\"packageUris\":[\"http://schema.mathworks.com/mf0/Connector/R2020b\"],\"version\":\"1.0\"}"
  G_motor_RR : Subsystem
      settings: PortSchema="{\"entries\":[{\"content\":{\"sides\":[{\"content\":{\"connectorIds\":[\"In1\",\"In2\"]},\"type\":\"ConnectorPlacement.EquallySpacedRectSide\",\"uuid\":\"b35581c9-4812-43f6-acf6-85982729658e\"},{\"content\":{\"connectorIds\":[\"Out1\"],\"side\":\"RIGHT\"},\"type\":\"ConnectorPlacement.EquallySpacedRectSide\",\"uuid\":\"46b9f9af-9e32-4108-a19f-3f2988ef12f0\"},{\"content\":{\"connectorIds\":[\"Out2\"],\"side\":\"TOP\"},\"type\":\"ConnectorPlacement.EquallySpacedRectSide\",\"uuid\":\"065300c1-2443-4807-8b2c-2500fecbac33\"}]},\"type\":\"ConnectorPlacement.EquallySpacedConnector\",\"uuid\":\"282786dd-8e40-401f-94f1-60a6482c0151\"}],\"packageUris\":[\"http://schema.mathworks.com/mf0/Connector/R2020b\"],\"version\":\"1.0\"}"
  Gain : Gain  Gain=7e4
  Gain12 : Gain  Gain=60*rid_ratio/(2*pi)
  Gain14 : Gain  Gain=R_wheel*3.6
  Gain7 : Gain  Gain=60*rid_ratio/(2*pi)
  Mux{,1..3} (4 alike) : Mux  Inputs=2
  eff_riduttore : Gain  Gain=rid_eff
  eff_riduttore2 : Gain  Gain=rid_eff
  ridut : Gain  Gain=rid_ratio
  ridut2 : Gain  Gain=rid_ratio
  derating : Outport
  Info Body : Outport  Port=2
  Vx[m/s] : Outport  Port=3
  Vy[m/s] : Outport  Port=4
  V[m/s] : Outport  Port=5
  Yaw : Outport  Port=6
  Yaw Rate : Outport  Port=7
  w_wheels [km/h] : Outport  Port=8
  Fz[N] : Outport  Port=9
  n_motor[rpm] : Outport  Port=10
  T_act : Outport  Port=11
  wires:
  eff_riduttore/1 -> ridut/1  "T_RR"
  Demux/4 -> Gain12/1
  Gain12/1 -> Mux2/2, G_motor_RR/2(rpm_motor)  "rpm"
  eff_riduttore2/1 -> ridut2/1  "T_RR"
  Car Body/8(omega [rad/s]) -> Gain14/1, Demux/1  "w"
  Gain7/1 -> Mux2/1, G_motor_RL/2(rpm_motor)  "rpm"
  G_motor_RR/1(T_out) -> Mux3/2, eff_riduttore2/1  "T_RR"
  G_motor_RL/1(T_out) -> Mux3/1, eff_riduttore/1  "T_RL"
  Demux/3 -> Gain7/1
  Steering Angle/1 -> Car Body/1(Steering Angle)
  ridut/1 -> Mux1/1
  T_req_RL/1 -> G_motor_RL/1(T_req)
  Mux1/1 -> Car Body/3(Torques)
  ridut2/1 -> Mux1/2
  T_req_RR/1 -> G_motor_RR/1(T_req)
  Brake %/1 -> Gain/1
  G_motor_RL/2(derating) -> Mux/1  "der_RL"
  G_motor_RR/2(derating) -> Mux/2  "der_RR"
  Mux/1 -> derating/1
  Gain/1 -> Car Body/2(Brake Pressure)  "brake Pa"
  Gain14/1 -> w_wheels [km/h]/1  "w_wheels [km/h]"
  Car Body/1(Info Body) -> Info Body/1
  Car Body/2(Vx[m/s]) -> Vx[m/s]/1  "vx"
  Car Body/3(Vy[m/s]) -> Vy[m/s]/1  "vy"
  Car Body/4(V[m/s]) -> V[m/s]/1
  Car Body/5(Yaw) -> Yaw/1  "yaw"
  Car Body/6(Yaw Rate) -> Yaw Rate/1
  Car Body/7(Fz) -> Fz[N]/1
  Mux2/1 -> n_motor[rpm]/1
  Mux3/1 -> T_act/1
